simulink model "Simulink"  (R2020b)
settings: Solver=ode45  StartTime=0.0  StopTime=30  FixedStep=0.01  MaxStep=0.001  RelTol=1e-6  AbsTol=1e-20
values from neighbouring files (symbols this model uses):
  A = [0 1;0 0]    [main.m]
  alpha = sqrt(alpha_2)    [main.m]
  B = [0;1]    [main.m]
  C = [1 1]    [main.m]
  c0 = Cc(1)    [main.m]
  c1 = sigma*ep/(2*norm(P2*B*B'*P2))    [main.m]
  c2 = ep0/(2*norm(P2*B*B'*P2))    [main.m]
  eta = 0.1    [main.m]
  F = Ac(:,1)    [main.m]
  H = P\Y    [main.m]
  L_kron_eye2 = kron(L,eye(2))    [main.m]
  L_kron_K = kron(L,K)    [main.m]
  M_kron_eye2 = kron(M,eye(2))    [main.m]
  mui = 0.4    [main.m]
  on_off = 0    [main.m]
  s = sqrt(0.1)    [main.m]
  Td = 0    [main.m]
  TITA = [1 1;0 -1]    [main.m]
  x1_0 = [1;2]    [main.m]
  x2_0 = [-1;2]    [main.m]
  x3_0 = [3;-2]    [main.m]
  x4_0 = [-2;3]    [main.m]
  x5_0 = [6;0]    [main.m]
libraries: simulink x6
settings Model: Creator=sokra  LastModifiedBy=sokra
settings SolverCC: AutoScaleAbsTol=off  ZeroCrossAlgorithm=Adaptive
settings DebuggingCC: IgnoredZcDiagnostic=none

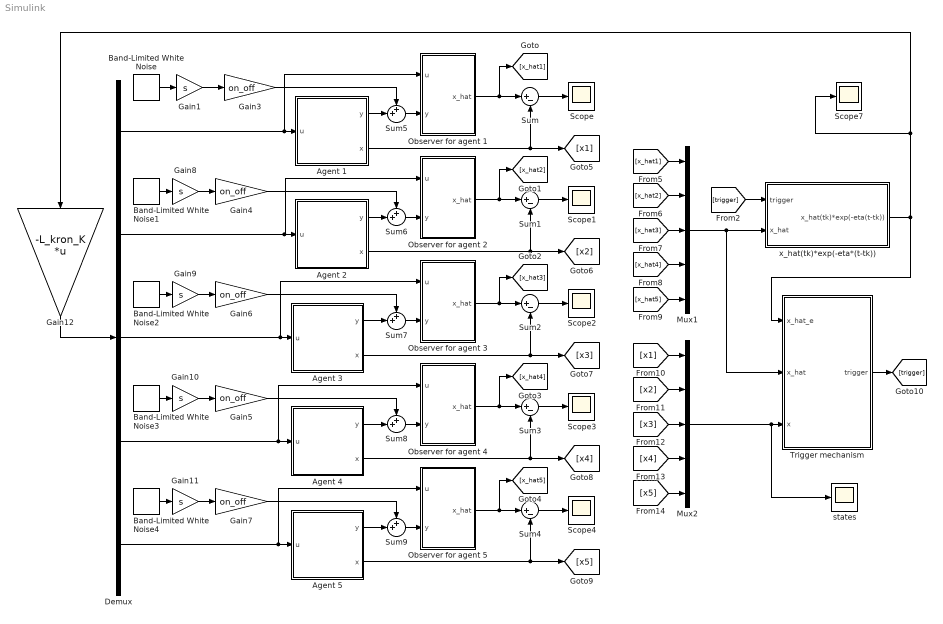
== system Simulink ==
  Agent 1 : Subsystem  mask{x0=x1_0}
  Agent 2 : Subsystem  mask{x0=x2_0}
  Agent 3 : Subsystem  mask{x0=x3_0}
  Agent 4 : Subsystem  mask{x0=x4_0}
  Agent 5 : Subsystem  mask{x0=x5_0}
  Band-Limited White Noise : simulink/Sources/Band-Limited White Noise  Cov=[1]  Ts=0.01  seed=[0]
  Band-Limited White Noise1 : simulink/Sources/Band-Limited White Noise  Cov=[1]  Ts=0.01  seed=[1]
  Band-Limited White Noise2 : simulink/Sources/Band-Limited White Noise  Cov=[1]  Ts=0.01  seed=[2]
  Band-Limited White Noise3 : simulink/Sources/Band-Limited White Noise  Cov=[1]  Ts=0.01  seed=[3]
  Band-Limited White Noise4 : simulink/Sources/Band-Limited White Noise  Cov=[1]  Ts=0.01  seed=[4]
  Demux : Demux  Outputs=5
  Gain{1,8..11} (5 alike) : Gain  Gain=s
  Gain12 : Gain  Gain=-L_kron_K  Multiplication=Matrix(K*u)
  Gain{3..7} (5 alike) : Gain  Gain=on_off
  Mux1 : Mux  Inputs=5
  Mux2 : Mux  Inputs=5
  Observer for agent 1 : Subsystem
  Observer for agent 2 : Subsystem
  Observer for agent 3 : Subsystem
  Observer for agent 4 : Subsystem
  Observer for agent 5 : Subsystem
  Scope{,1..4,7} (6 alike) : Scope
  Sum{,1..4} (5 alike) : Sum  Inputs=|+-
  Sum{5..9} (5 alike) : Sum  Inputs=++|
  Trigger mechanism : Subsystem
  states : Scope
  x_hat(tk)*exp(-eta*(t-tk)) : Subsystem
  wires:
  Gain7/1 -> Sum9/1
  Sum7/1 -> Observer for agent 3/2(y)
  Sum8/1 -> Observer for agent 4/2(y)
  Sum9/1 -> Observer for agent 5/2(y)
  Agent 2/2(x) -> [x2], Sum1/2
  [x_hat2] -> Mux1/2
  Gain4/1 -> Sum6/1
  Sum5/1 -> Observer for agent 1/2(y)
  Sum6/1 -> Observer for agent 2/2(y)
  Agent 5/1(y) -> Sum9/2
  Mux2/1 -> states/1, Trigger mechanism/3(x)
  [x4] -> Mux2/4
  Trigger mechanism/1(trigger) -> [trigger]
  Gain3/1 -> Sum5/1
  Agent 2/1(y) -> Sum6/2
  [x_hat4] -> Mux1/4
  Observer for agent 3/1(x_hat) -> [x_hat3], Sum2/1
  Gain5/1 -> Sum8/1
  Agent 3/1(y) -> Sum7/2
  Observer for agent 5/1(x_hat) -> [x_hat5], Sum4/1
  [x_hat5] -> Mux1/5
  Agent 1/1(y) -> Sum5/2
  Agent 4/1(y) -> Sum8/2
  Band-Limited White Noise/1 -> Gain1/1
  Gain6/1 -> Sum7/1
  [x3] -> Mux2/3
  Agent 4/2(x) -> [x4], Sum3/2
  Gain12/1 -> Demux/1
  Mux1/1 -> x_hat(tk)*exp(-eta*(t-tk))/2(x_hat), Trigger mechanism/2(x_hat)
  [x2] -> Mux2/2
  Observer for agent 2/1(x_hat) -> [x_hat2], Sum1/1
  Sum4/1 -> Scope4/1
  [x_hat3] -> Mux1/3
  Agent 5/2(x) -> [x5], Sum4/2
  [trigger] -> x_hat(tk)*exp(-eta*(t-tk))/1(trigger)
  x_hat(tk)*exp(-eta*(t-tk))/1(x_hat(tk)*exp(-eta(t-tk))) -> Scope7/1, Gain12/1, Trigger mechanism/1(x_hat_e)
  Agent 1/2(x) -> [x1], Sum/2
  Agent 3/2(x) -> [x3], Sum2/2
  Observer for agent 1/1(x_hat) -> [x_hat1], Sum/1
  [x5] -> Mux2/5
  Observer for agent 4/1(x_hat) -> [x_hat4], Sum3/1
  Sum1/1 -> Scope1/1
  Sum3/1 -> Scope3/1
  Sum/1 -> Scope/1
  [x1] -> Mux2/1
  [x_hat1] -> Mux1/1
  Sum2/1 -> Scope2/1
  Demux/1 -> Agent 1/1(u), Observer for agent 1/1(u)
  Demux/2 -> Agent 2/1(u), Observer for agent 2/1(u)
  Demux/3 -> Agent 3/1(u), Observer for agent 3/1(u)
  Demux/4 -> Agent 4/1(u), Observer for agent 4/1(u)
  Demux/5 -> Agent 5/1(u), Observer for agent 5/1(u)
  Gain1/1 -> Gain3/1
  Band-Limited White Noise1/1 -> Gain8/1
  Gain8/1 -> Gain4/1
  Gain9/1 -> Gain6/1
  Band-Limited White Noise2/1 -> Gain9/1
  Band-Limited White Noise3/1 -> Gain10/1
  Gain10/1 -> Gain5/1
  Gain11/1 -> Gain7/1
  Band-Limited White Noise4/1 -> Gain11/1

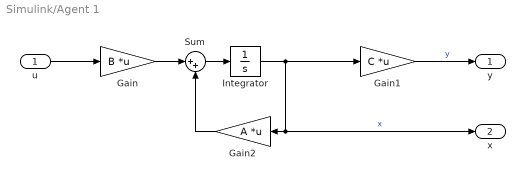
== system Simulink/Agent 1 ==
  u : Inport
  Gain : Gain  Gain=B  Multiplication=Matrix(K*u)
  Gain1 : Gain  Gain=C  Multiplication=Matrix(K*u)
  Gain2 : Gain  Gain=A  Multiplication=Matrix(K*u)
  Integrator : Integrator  InitialCondition=x0
  Sum : Sum  Inputs=|++
  y : Outport
  x : Outport  Port=2
  wires:
  Sum/1 -> Integrator/1
  Integrator/1 -> x/1, Gain2/1, Gain1/1  "x"
  u/1 -> Gain/1
  Gain/1 -> Sum/1
  Gain2/1 -> Sum/2
  Gain1/1 -> y/1  "y"

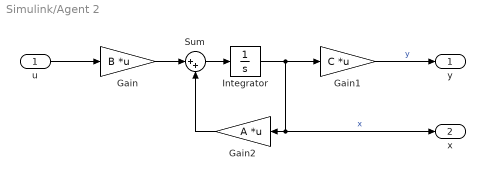
== system Simulink/Agent 2 ==
  u : Inport
  Gain : Gain  Gain=B  Multiplication=Matrix(K*u)
  Gain1 : Gain  Gain=C  Multiplication=Matrix(K*u)
  Gain2 : Gain  Gain=A  Multiplication=Matrix(K*u)
  Integrator : Integrator  InitialCondition=x0
  Sum : Sum  Inputs=|++
  y : Outport
  x : Outport  Port=2
  wires:
  Gain1/1 -> y/1  "y"
  Gain2/1 -> Sum/2
  Gain/1 -> Sum/1
  u/1 -> Gain/1
  Sum/1 -> Integrator/1
  Integrator/1 -> Gain1/1, x/1, Gain2/1  "x"

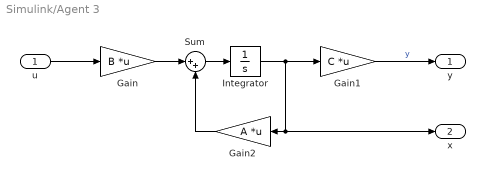
== system Simulink/Agent 3 ==
  u : Inport
  Gain : Gain  Gain=B  Multiplication=Matrix(K*u)
  Gain1 : Gain  Gain=C  Multiplication=Matrix(K*u)
  Gain2 : Gain  Gain=A  Multiplication=Matrix(K*u)
  Integrator : Integrator  InitialCondition=x0
  Sum : Sum  Inputs=|++
  y : Outport
  x : Outport  Port=2
  wires:
  Sum/1 -> Integrator/1
  Integrator/1 -> x/1, Gain2/1, Gain1/1
  u/1 -> Gain/1
  Gain/1 -> Sum/1
  Gain2/1 -> Sum/2
  Gain1/1 -> y/1  "y"

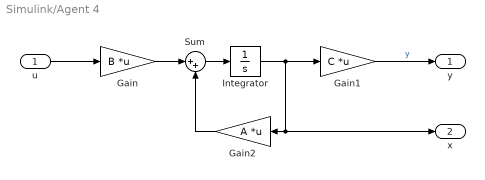
== system Simulink/Agent 4 ==
  u : Inport
  Gain : Gain  Gain=B  Multiplication=Matrix(K*u)
  Gain1 : Gain  Gain=C  Multiplication=Matrix(K*u)
  Gain2 : Gain  Gain=A  Multiplication=Matrix(K*u)
  Integrator : Integrator  InitialCondition=x0
  Sum : Sum  Inputs=|++
  y : Outport
  x : Outport  Port=2
  wires:
  Gain1/1 -> y/1  "y"
  Gain2/1 -> Sum/2
  Gain/1 -> Sum/1
  u/1 -> Gain/1
  Integrator/1 -> Gain1/1, x/1, Gain2/1
  Sum/1 -> Integrator/1

== system Simulink/Agent 5 ==
  u : Inport
  Gain : Gain  Gain=B  Multiplication=Matrix(K*u)
  Gain1 : Gain  Gain=C  Multiplication=Matrix(K*u)
  Gain2 : Gain  Gain=A  Multiplication=Matrix(K*u)
  Integrator : Integrator  InitialCondition=x0
  Sum : Sum  Inputs=|++
  y : Outport
  x : Outport  Port=2
  wires:
  Sum/1 -> Integrator/1
  Integrator/1 -> x/1, Gain2/1, Gain1/1
  u/1 -> Gain/1
  Gain/1 -> Sum/1
  Gain2/1 -> Sum/2
  Gain1/1 -> y/1  "y"

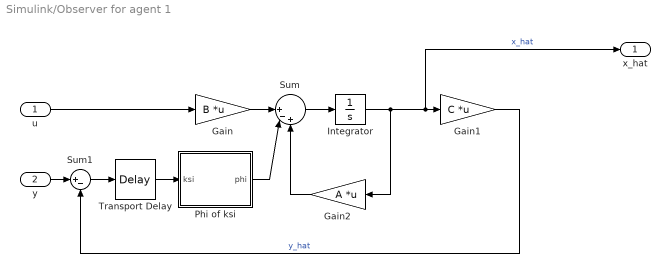
== system Simulink/Observer for agent 1 ==
  u : Inport
  y : Inport  Port=2
  Gain : Gain  Gain=B  Multiplication=Matrix(K*u)
  Gain1 : Gain  Gain=C  Multiplication=Matrix(K*u)
  Gain2 : Gain  Gain=A  Multiplication=Matrix(K*u)
  Integrator : Integrator  InitialCondition=[0;0]
  Phi of ksi : MATLAB Function  TreatAsAtomicUnit=on
  Sum : Sum  Inputs=||+-+
  Sum1 : Sum  Inputs=|+-
  Transport Delay : TransportDelay  DelayTime=Td
  x_hat : Outport
  wires:
  Gain/1 -> Sum/1
  Phi of ksi/1(phi) -> Sum/2
  Gain1/1 -> Sum1/2  "y_hat"
  Integrator/1 -> Gain2/1, x_hat/1, Gain1/1  "x_hat"
  Sum/1 -> Integrator/1
  y/1 -> Sum1/1
  u/1 -> Gain/1
  Gain2/1 -> Sum/3
  Sum1/1 -> Transport Delay/1
  Transport Delay/1 -> Phi of ksi/1(ksi)

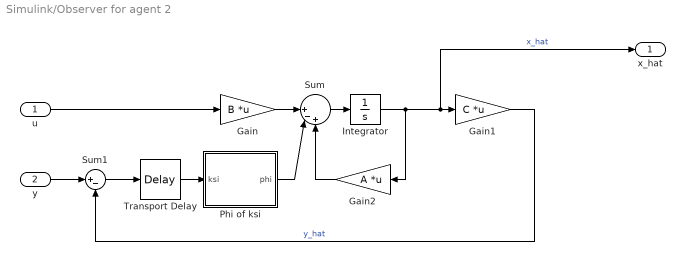
== system Simulink/Observer for agent 2 ==
  u : Inport
  y : Inport  Port=2
  Gain : Gain  Gain=B  Multiplication=Matrix(K*u)
  Gain1 : Gain  Gain=C  Multiplication=Matrix(K*u)
  Gain2 : Gain  Gain=A  Multiplication=Matrix(K*u)
  Integrator : Integrator  InitialCondition=[0;0]
  Phi of ksi : MATLAB Function  TreatAsAtomicUnit=on
  Sum : Sum  Inputs=||+-+
  Sum1 : Sum  Inputs=|+-
  Transport Delay : TransportDelay  DelayTime=Td
  x_hat : Outport
  wires:
  u/1 -> Gain/1
  Integrator/1 -> Gain1/1, x_hat/1, Gain2/1  "x_hat"
  Sum/1 -> Integrator/1
  Gain2/1 -> Sum/3
  Sum1/1 -> Transport Delay/1
  Gain1/1 -> Sum1/2  "y_hat"
  Phi of ksi/1(phi) -> Sum/2
  y/1 -> Sum1/1
  Gain/1 -> Sum/1
  Transport Delay/1 -> Phi of ksi/1(ksi)

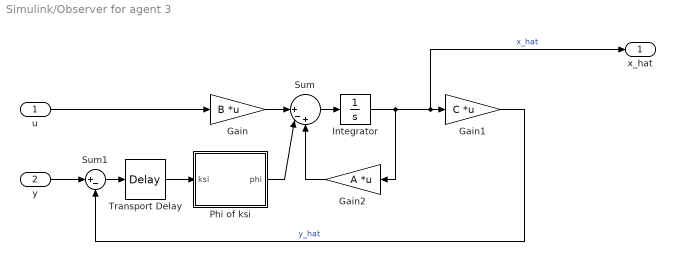
== system Simulink/Observer for agent 3 ==
  u : Inport
  y : Inport  Port=2
  Gain : Gain  Gain=B  Multiplication=Matrix(K*u)
  Gain1 : Gain  Gain=C  Multiplication=Matrix(K*u)
  Gain2 : Gain  Gain=A  Multiplication=Matrix(K*u)
  Integrator : Integrator  InitialCondition=[0;0]
  Phi of ksi : MATLAB Function  TreatAsAtomicUnit=on
  Sum : Sum  Inputs=||+-+
  Sum1 : Sum  Inputs=|+-
  Transport Delay : TransportDelay  DelayTime=Td
  x_hat : Outport
  wires:
  Gain/1 -> Sum/1
  y/1 -> Sum1/1
  Phi of ksi/1(phi) -> Sum/2
  Gain1/1 -> Sum1/2  "y_hat"
  Sum1/1 -> Transport Delay/1
  Gain2/1 -> Sum/3
  Sum/1 -> Integrator/1
  Integrator/1 -> Gain2/1, x_hat/1, Gain1/1  "x_hat"
  u/1 -> Gain/1
  Transport Delay/1 -> Phi of ksi/1(ksi)

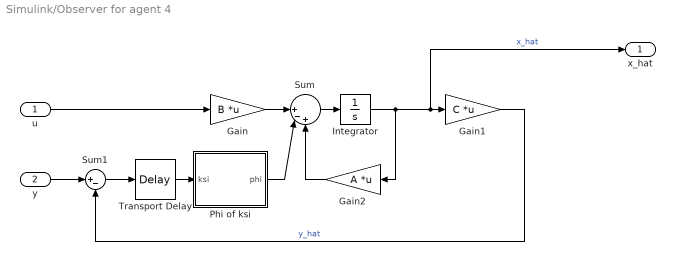
== system Simulink/Observer for agent 4 ==
  u : Inport
  y : Inport  Port=2
  Gain : Gain  Gain=B  Multiplication=Matrix(K*u)
  Gain1 : Gain  Gain=C  Multiplication=Matrix(K*u)
  Gain2 : Gain  Gain=A  Multiplication=Matrix(K*u)
  Integrator : Integrator  InitialCondition=[0;0]
  Phi of ksi : MATLAB Function  TreatAsAtomicUnit=on
  Sum : Sum  Inputs=||+-+
  Sum1 : Sum  Inputs=|+-
  Transport Delay : TransportDelay  DelayTime=Td
  x_hat : Outport
  wires:
  u/1 -> Gain/1
  Integrator/1 -> Gain1/1, x_hat/1, Gain2/1  "x_hat"
  Sum/1 -> Integrator/1
  Gain2/1 -> Sum/3
  Sum1/1 -> Transport Delay/1
  Gain1/1 -> Sum1/2  "y_hat"
  Phi of ksi/1(phi) -> Sum/2
  y/1 -> Sum1/1
  Gain/1 -> Sum/1
  Transport Delay/1 -> Phi of ksi/1(ksi)

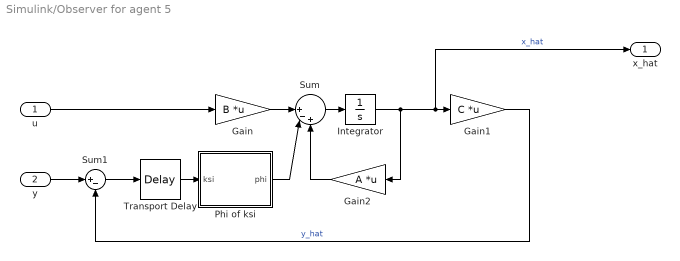
== system Simulink/Observer for agent 5 ==
  u : Inport
  y : Inport  Port=2
  Gain : Gain  Gain=B  Multiplication=Matrix(K*u)
  Gain1 : Gain  Gain=C  Multiplication=Matrix(K*u)
  Gain2 : Gain  Gain=A  Multiplication=Matrix(K*u)
  Integrator : Integrator  InitialCondition=[0;0]
  Phi of ksi : MATLAB Function  TreatAsAtomicUnit=on
  Sum : Sum  Inputs=||+-+
  Sum1 : Sum  Inputs=|+-
  Transport Delay : TransportDelay  DelayTime=Td
  x_hat : Outport
  wires:
  Gain/1 -> Sum/1
  y/1 -> Sum1/1
  Phi of ksi/1(phi) -> Sum/2
  Gain1/1 -> Sum1/2  "y_hat"
  Sum1/1 -> Transport Delay/1
  Gain2/1 -> Sum/3
  Sum/1 -> Integrator/1
  Integrator/1 -> Gain2/1, x_hat/1, Gain1/1  "x_hat"
  u/1 -> Gain/1
  Transport Delay/1 -> Phi of ksi/1(ksi)

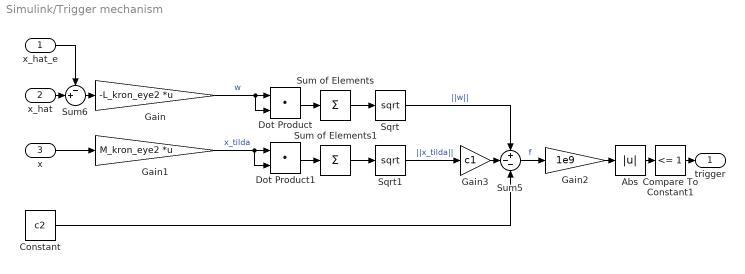
== system Simulink/Trigger mechanism ==
  x_hat_e : Inport
  x_hat : Inport  Port=2
  x : Inport  Port=3
  Abs : Abs
  Compare To Constant1 : simulink/Logic and Bit Operations/Compare To Constant  relop=<=  const=1  OutDataTypeStr=boolean
  Constant : Constant  Value=c2
  Dot Product : DotProduct  InputSameDT=on  OutDataTypeStr=Inherit: Inherit via internal rule
  Dot Product1 : DotProduct  InputSameDT=on  OutDataTypeStr=Inherit: Inherit via internal rule
  Gain : Gain  Gain=-L_kron_eye2  Multiplication=Matrix(K*u)
  Gain1 : Gain  Gain=M_kron_eye2  Multiplication=Matrix(K*u)
  Gain2 : Gain  Gain=1e9
  Gain3 : Gain  Gain=c1
  Sqrt : Sqrt  SaturateOnIntegerOverflow=on
  Sqrt1 : Sqrt  SaturateOnIntegerOverflow=on
  Sum of Elements : Sum  Inputs=+
  Sum of Elements1 : Sum  Inputs=+
  Sum5 : Sum  Inputs=+--
  Sum6 : Sum  Inputs=-+|
  trigger : Outport
  wires:
  Sum of Elements/1 -> Sqrt/1
  Constant/1 -> Sum5/3
  Gain1/1 -> Dot Product1/2, Dot Product1/1  "x_tilda"
  Sum5/1 -> Gain2/1  "f"
  Gain3/1 -> Sum5/2
  Dot Product/1 -> Sum of Elements/1
  Gain/1 -> Dot Product/2, Dot Product/1  "w"
  Dot Product1/1 -> Sum of Elements1/1
  Sum of Elements1/1 -> Sqrt1/1
  Sum6/1 -> Gain/1
  Sqrt1/1 -> Gain3/1  "||x_tilda||"
  Sqrt/1 -> Sum5/1  "||w||"
  x_hat/1 -> Sum6/2
  x_hat_e/1 -> Sum6/1
  x/1 -> Gain1/1
  Gain2/1 -> Abs/1
  Abs/1 -> Compare To Constant1/1
  Compare To Constant1/1 -> trigger/1

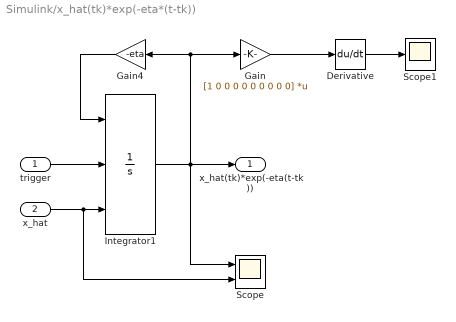
== system Simulink/x_hat(tk)*exp(-eta*(t-tk)) ==
  trigger : Inport
  x_hat : Inport  Port=2
  Derivative : Derivative
  Gain : Gain  Gain=[1 0 0 0 0 0 0 0 0 0]  Multiplication=Matrix(K*u)
  Gain4 : Gain  Gain=-eta
  Integrator1 : Integrator  ExternalReset=level  InitialConditionSource=external
  Scope : Scope  NumInputPorts=2
  Scope1 : Scope
  x_hat(tk)*exp(-eta(t-tk)) : Outport
  wires:
  Gain4/1 -> Integrator1/1
  Integrator1/1 -> Gain4/1, Gain/1, Scope/1, x_hat(tk)*exp(-eta(t-tk))/1
  trigger/1 -> Integrator1/2
  x_hat/1 -> Scope/2, Integrator1/3
  Derivative/1 -> Scope1/1
  Gain/1 -> Derivative/1

== matlab function Simulink/Observer for agent 2/Phi of ksi ==
  data: ksi input; phi output double size=2; c0 parameter; alpha parameter; TITA parameter; mui parameter; H parameter; F parameter
function phi = fcn(ksi,c0, alpha, TITA, mui, H, F)
if(ksi~=0)
    x=abs(c0)/alpha./abs(ksi);
    phi=TITA\([x^(mui/(1+mui)) 0;0 x^(2*mui/(1+mui))]*H-F)*ksi/c0;
else 
    phi=[0;0];
end

== matlab function Simulink/Observer for agent 3/Phi of ksi ==
  data: ksi input; phi output double size=2; c0 parameter; alpha parameter; TITA parameter; mui parameter; H parameter; F parameter
function phi = fcn(ksi,c0, alpha, TITA, mui, H, F)
if(ksi~=0)
    x=abs(c0)/alpha./abs(ksi);
    phi=TITA\([x^(mui/(1+mui)) 0;0 x^(2*mui/(1+mui))]*H-F)*ksi/c0;
else 
    phi=[0;0];
end

== matlab function Simulink/Observer for agent 4/Phi of ksi ==
  data: ksi input; phi output double size=2; c0 parameter; alpha parameter; TITA parameter; mui parameter; H parameter; F parameter
function phi = fcn(ksi,c0, alpha, TITA, mui, H, F)
if(ksi~=0)
    x=abs(c0)/alpha./abs(ksi);
    phi=TITA\([x^(mui/(1+mui)) 0;0 x^(2*mui/(1+mui))]*H-F)*ksi/c0;
else 
    phi=[0;0];
end

== matlab function Simulink/Observer for agent 5/Phi of ksi ==
  data: ksi input; phi output double size=2; c0 parameter; alpha parameter; TITA parameter; mui parameter; H parameter; F parameter
function phi = fcn(ksi,c0, alpha, TITA, mui, H, F)
if(ksi~=0)
    x=abs(c0)/alpha./abs(ksi);
    phi=TITA\([x^(mui/(1+mui)) 0;0 x^(2*mui/(1+mui))]*H-F)*ksi/c0;
else 
    phi=[0;0];
end

== matlab function Simulink/Observer for agent 1/Phi of ksi ==
  data: ksi input; phi output double size=2; c0 parameter; alpha parameter; TITA parameter; mui parameter; H parameter; F parameter
function phi = fcn(ksi,c0, alpha, TITA, mui, H, F)
if(ksi~=0)
    x=abs(c0)/alpha./abs(ksi);
    phi=TITA\([x^(mui/(1+mui)) 0;0 x^(2*mui/(1+mui))]*H-F)*ksi/c0;
else 
    phi=[0;0];
end
